simulink model "simL0_multiPath"  (R2024a)
settings: Solver=ode4  StartTime=0.0  StopTime=1500  FixedStep=0.01  MaxStep=0.01  MinStep=10^-3  RelTol=0.01
values from neighbouring files (symbols this model uses):
  MegAWESkite = yaml.ReadYaml('MegAWESkite.yaml',false,true)    [runMain.m]
undefined symbols (not defined in the file or in its folder): actuatorLimit, controllerGains_retraction, controllerGains_traction, DiscIntNeverNeededParam, ENVMT, pathparam, simInit, tetherParams, winchParameter
libraries: simulink x9, slpidlib x9, sharedtransform x3, aerolibutil x3, dspswit3 x2, dspinverses x2, shared6dof x1, simulink_extras x1, dspsigops x1, dspstat3 x1, vrlib x1
(part 1 of 5)
settings Model: Creator=Gian  LastModifiedBy=dylaneijkelhof
settings SolverCC: MaxConsecutiveMinStep=1000000000  AlgebraicLoopSolver=LineSearch  MinimalZcImpactIntegration=on
settings DataIOCC: SaveOperatingPoint=on  SaveOutput=off  SignalLogging=off  DSMLogging=off  SaveTime=off
settings OptimizationCC: LifeSpan=inf
settings DebuggingCC: ReadBeforeWriteMsg=DisableAll  WriteAfterWriteMsg=DisableAll  WriteAfterReadMsg=DisableAll  MultiTaskDSMMsg=none  MultiTaskRateTransMsg=warning  UnconnectedInputMsg=warning  UnconnectedOutputMsg=warning  UnconnectedLineMsg=warning  SFUnexpectedBacktrackingDiag=warning  SFNoUnconditionalDefaultTransitionDiag=warning  SFExecutionAtInitializationDiag=none  ArithmeticOperatorsInVariantConditions=warning
settings ModelReferenceCC: UpdateModelReferenceTargets=IfOutOfDate  EnableRefExpFcnMdlSchedulingChecks=on  ModelReferenceMinAlgLoopOccurrences=on
settings SFSimCC: SFSimEcho=off  SimUseLocalCustomCode=off  CustomCodeUndefinedFunction=UseInterfaceOnly
settings RTWCC: RTWUseLocalCustomCode=off  GPUComputeCapability=3.5
settings CodeAppCC: StateflowObjectComments=on
settings GRTTargetCC: TargetLangStandard=C89/C90 (ANSI)
settings ConfigComp: CovMetricSettings=dw  CovSaveCumulativeToWorkspaceVar=on  CovSaveSingleToWorkspaceVar=on  CovExternalEMLEnable=off

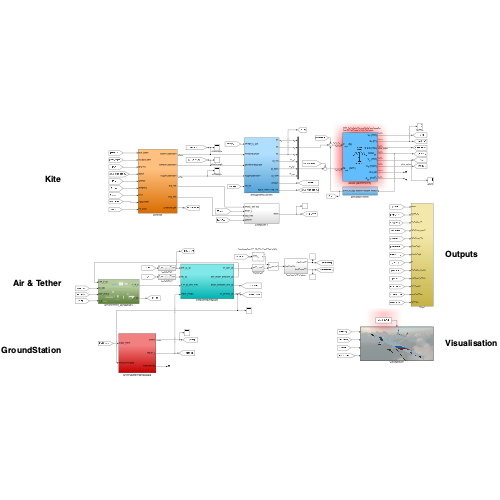
[thumbnail: Simulink's stored preview of the top-level diagram]
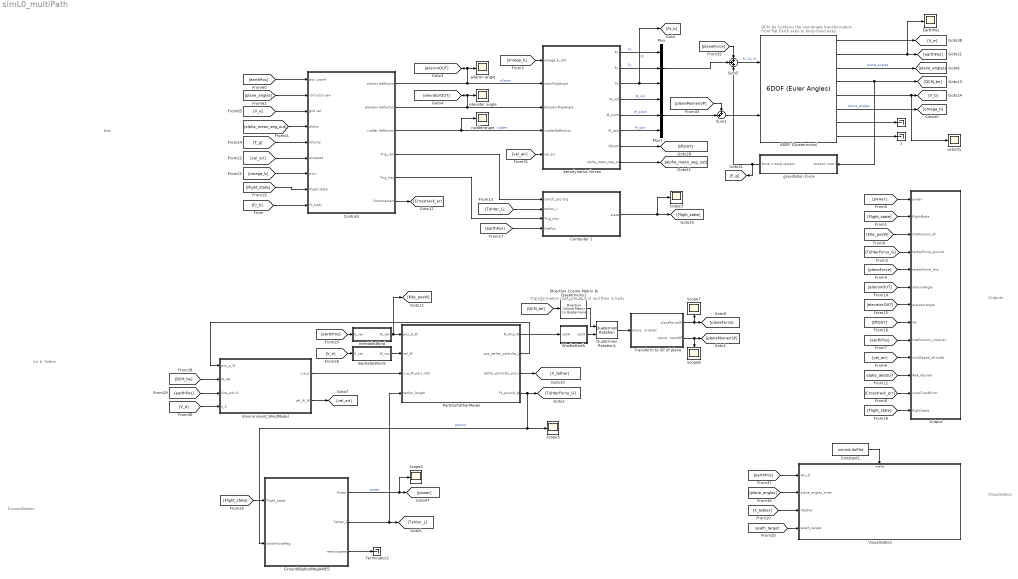
== system simL0_multiPath ==
  note: GroundStation
  note: Transformation of Ft_kite W in O and then in body
  note: DCM_be Contains the coordinate transformation
      | from flat Earth axes to body-fixed axes.
  note: Air & Tether
  note: Kite
  note: Outputs
  note: Visualisation
  "  " : Terminator
  "  1" : Terminator
  6DOF (Quaternions) : shared6dof/6DOF (Euler Angles)  units=Metric (MKS)  mtype=Fixed  rep=Quaternion  xme_0=simInit.pos_O_init  Vm_0=simInit.iniVel  eul_0=simInit.iniEul  pm_0=simInit.bodyRotationRates_init  mass_0=MegAWESkite.mass_aircraft  mass_e=0.5  mass_f=2.0  inertia=MegAWESkite.I_aircraft  inertia_e=eye(3)  inertia_f=2*eye(3)  k_quat=1.0  vre_flag=on  abi_flag=off  aMode=aMode  xme_statename=''  Vm_statename=''  eul_statename=''  quat_statename=''  pm_statename=''  mass_statename=''
  Computer 1 : Subsystem
  Constant1 : Constant  Value=simInit.doPlot
  Controls : Subsystem
  Direction Cosine Matrix to Quaternions1 : sharedtransform/Direction Cosine Matrix  to Quaternions  aMode=aMode  action=None  tolerance=eps(2)
  EarthPos : Scope
  Environment_WindModel : Subsystem
  GroundStationMegAWES : Subsystem
  InertialtoWind : Subsystem
  InertialtoWind1 : Subsystem
  Mux : Mux  Inputs=3
  Mux1 : Mux  Inputs=3
  Output : Subsystem
  ParticleTetherModel : Subsystem
  Quaternion Rotation1 : aerolibutil/Quaternion Rotation
  Scope{2..3,5,7..8} (5 alike) : Scope
  Sum1 : Sum  Inputs=++|
  Sum5 : Sum  Inputs=+++
  Terminator2 : Terminator
  Transform to SP of plane : Subsystem
  Visualisation : Subsystem
      mask Display: image('/Users/dylaneijkelhof/Documents/Matlab/MegAWES/Lib/DE2019_Aircraft.jpeg'); % Use "Edit Image" on toolstrip to change.
  WindtoEarth : Subsystem
  aerodynamic forces : Subsystem
  aileron angle : Scope
  elevator angle : Scope
  gravitation force : Subsystem
  rudderangle : Scope
  velocity : Scope
  wires:
  6DOF (Quaternions)/7 -> "  "/1
  6DOF (Quaternions)/4 -> gravitation force/1(rotation matrix), [DCM_be]
  6DOF (Quaternions)/5 -> velocity/1, [V_b]
  6DOF (Quaternions)/3 -> [plane_angles]  "plane_angles"
  aerodynamic forces/5(M_pitch) -> Mux1/2  "M_pitch"
  aerodynamic forces/6(M_yaw) -> Mux1/3  "M_yaw"
  aerodynamic forces/2(Fy) -> Mux/2  "Fy"
  aerodynamic forces/3(Fz) -> Mux/3, [Fz_b]  "Fz"
  aerodynamic forces/4(M_roll) -> Mux1/1  "M_roll"
  aerodynamic forces/1(Fx) -> Mux/1  "Fx"
  Mux/1 -> Sum5/2
  gravitation force/1(force in body system) -> Sum5/3, [F_g]
  Sum5/1 -> 6DOF (Quaternions)/1  "Fx, Fy, Fz"
  Controls/1(aileron deflection) -> [aileronOUT], aileron angle/1, aerodynamic forces/2(mainFlapAngle)  "aileron"
  Mux1/1 -> Sum1/2
  Sum1/1 -> 6DOF (Quaternions)/2
  6DOF (Quaternions)/1 -> [V_e]
  6DOF (Quaternions)/6 -> [omega_b]  "plane_angles"
  aerodynamic forces/7(liftOUT) -> [liftOUT]
  aerodynamic forces/8(alpha_mean_seg_out) -> [alpha_mean_seg_out]
  [earthPos] -> Controls/1("pos. plane ")
  [plane_angles] -> Controls/2(roll pitch yaw)
  [V_e] -> Controls/3(gnd vel.)
  [alpha_mean_seg_out] -> Controls/4(alpha)
  [vel_air] -> Controls/6(airspeed)
  [omega_b] -> Controls/7(p-q-r)
  [F_g] -> Controls/5(Gravity)
  6DOF (Quaternions)/8 -> "  1"/1
  [omega_b] -> aerodynamic forces/1(omega_b_dist)
  [Fz_b] -> Controls/9("Fz_body ")
  GroundStationMegAWES/3(reeloutspeed) -> Terminator2/1
  6DOF (Quaternions)/2 -> EarthPos/1, [earthPos]
  GroundStationMegAWES/1(Power) -> Scope2/1, [power]  "power"
  Controls/2(elevator deflection) -> aerodynamic forces/3(ElevatorFlapAngle), [elevatorOUT], elevator angle/1
  [Flight_state] -> Controls/8(Flight state)
  [Flight_state] -> GroundStationMegAWES/1(Flight_state)
  ParticleTetherModel/2(pos_tether_particles_W) -> Environment_WindModel/1(pos_p_W)
  [earthPos] -> InertialtoWind/1(E_vec)
  InertialtoWind/1(W_vec) -> [Kite_posW], ParticleTetherModel/1(pos_G_W)
  InertialtoWind1/1(W_vec) -> ParticleTetherModel/2(vel_W)
  [V_e] -> InertialtoWind1/1(E_vec)
  Environment_WindModel/1(v_w_p) -> ParticleTetherModel/3(v_w_W_part_mat)
  GroundStationMegAWES/2(Tether_L) -> ParticleTetherModel/4(tether_length), [Tehter_L]
  [DCM_be] -> Environment_WindModel/2(M_OB)
  [earthPos] -> Environment_WindModel/3(Kite_pos O)
  Environment_WindModel/2(vel_W_W) -> [vel_air]
  [V_b] -> Environment_WindModel/4(v_b)
  Transform to SP of plane/2(planeMomentSP) -> [planeMomenSP], Scope8/1
  Transform to SP of plane/1(planeForceSP) -> [planeForce], Scope7/1
  [vel_air] -> aerodynamic forces/5(vel_air)
  [planeForce] -> Sum5/1
  ParticleTetherModel/4(Ft_ground_W) -> GroundStationMegAWES/2(winchForceMag), Scope5/1, [TehterForce_G]  "ground"
  ParticleTetherModel/1(Ft_Kite_W) -> WindtoEarth/1(vecW)
  Direction Cosine Matrix to Quaternions1/1 -> Quaternion Rotation1/1
  [DCM_be] -> Direction Cosine Matrix to Quaternions1/1
  WindtoEarth/1(vecO) -> Quaternion Rotation1/2
  Quaternion Rotation1/1 -> Transform to SP of plane/1(planeForceVec)
  [planeMomenSP] -> Sum1/1
  ParticleTetherModel/3(tether_particles_pos_W) -> [X_tether]
  [X_tether] -> Visualisation/3(Xtether)
  [plane_angles] -> Visualisation/2(plane_angles_euler)
  [earthPos] -> Visualisation/1(Pos_O)
  Controls/3(rudder deflection) -> rudderangle/1, aerodynamic forces/4(rudderDeflection)  "rudder"
  Controls/6(Crosstrackerr) -> [Crosstrack_err]
  Controls/4(Trig_retr) -> Computer 1/1(switch_pos trig)
  Computer 1/1(state) -> Scope3/1, [Flight_state]
  Controls/5(Trig_trac) -> Computer 1/3(Trig_trac)
  [Tehter_L] -> Computer 1/2(tether_L)
  [earthPos] -> Computer 1/4(kitePos)
  Constant1/1 -> Visualisation/Enable
  [spath_target] -> Visualisation/4(spath_target)
  [Flight_state] -> Output/2(flightMode)
  [Kite_posW] -> Output/3(kitePosition_W)
  [TehterForce_G] -> Output/4(tetherForce_ground)
  [planeForce] -> Output/5(tetherForce_kite)
  [aileronOUT] -> Output/6(aileronAngle)
  [elevatorOUT] -> Output/7(elevatorAngle)
  [liftOUT] -> Output/8(lift)
  [earthPos] -> Output/9(kitePosition_intertial)
  [vel_air] -> Output/10(windSpeed_altitude)
  [alpha_desOUT] -> Output/11(AoA_desired)
  [Crosstrack_err] -> Output/12(crossTrackError)
  [Flight_state] -> Output/13(flightState)
  [power] -> Output/1(power)

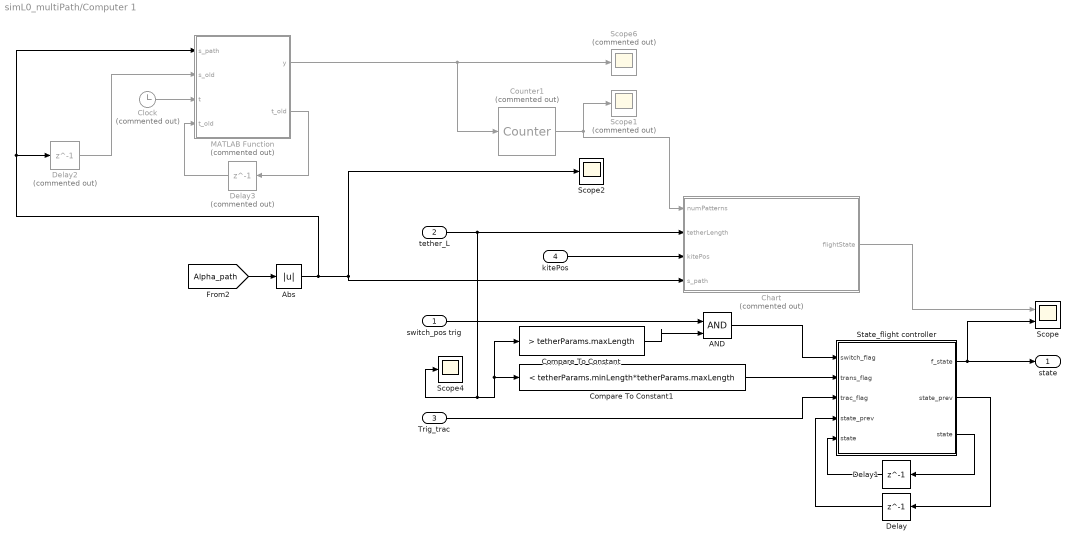
== system simL0_multiPath/Computer 1 ==
  switch_pos trig : Inport
  tether_L : Inport  Port=2
  Trig_trac : Inport  Port=3
  kitePos : Inport  Port=4
  AND : Logic  IconShape=distinctive  AllPortsSameDT=off  OutDataTypeStr=boolean
  Abs : Abs  SaturateOnIntegerOverflow=off
  Chart : Stateflow chart  Commented=on  TreatAsAtomicUnit=on
  Clock : Clock  Commented=on
  Compare To Constant : simulink/Logic and Bit Operations/Compare To Constant  relop=>  const=tetherParams.maxLength  OutDataTypeStr=boolean
  Compare To Constant1 : simulink/Logic and Bit Operations/Compare To Constant  relop=<  const=tetherParams.minLength*tetherParams.maxLength  OutDataTypeStr=boolean
  Counter1 : dspswit3/Counter  Commented=on  Direction=Up  CountEvent=Non-zero sample  CounterSize=User defined  MaxCount=1e9  InitialCount=0  Output=Count  HitValue=32  ResetInput=off  SamplesPerFrame=1  Ts=1  CntDtype=double  HitDtype=Logical
  Delay : Delay  DelayLength=1  InitialCondition=1
  Delay1 : Delay  DelayLength=1  InitialCondition=1
  Delay2 : Delay  Commented=on  DelayLength=1
  Delay3 : Delay  Commented=on  DelayLength=1
  MATLAB Function : MATLAB Function  Commented=on  TreatAsAtomicUnit=on
  Scope : Scope  NumInputPorts=2
  Scope1 : Scope  Commented=on
  Scope2 : Scope
  Scope4 : Scope
  Scope6 : Scope  Commented=on
  State_flight controller : MATLAB Function  TreatAsAtomicUnit=on
  state : Outport
  wires:
  tether_L/1 -> Scope4/1, Compare To Constant/1, Compare To Constant1/1, Chart/2(tetherLength)
  AND/1 -> State_flight controller/1(switch_flag)
  Compare To Constant1/1 -> State_flight controller/2(trans_flag)
  switch_pos trig/1 -> AND/1
  State_flight controller/1(f_state) -> Scope/2, state/1
  Compare To Constant/1 -> AND/2
  Trig_trac/1 -> State_flight controller/3(trac_flag)
  Chart/1(flightState) -> Scope/1
  kitePos/1 -> Chart/3(kitePos)
  [Alpha_path] -> Abs/1
  Delay/1 -> State_flight controller/4("state_prev ")
  State_flight controller/2(state_prev) -> Delay/1
  Delay1/1 -> State_flight controller/5("state ")
  State_flight controller/3(state) -> Delay1/1
  Abs/1 -> MATLAB Function/1(s_path), Delay2/1, Scope2/1, Chart/4(s_path)
  Counter1/1 -> Chart/1(numPatterns), Scope1/1
  Delay2/1 -> MATLAB Function/2(s_old)
  MATLAB Function/1(y) -> Counter1/1, Scope6/1
  MATLAB Function/2(t_old) -> Delay3/1
  Delay3/1 -> MATLAB Function/4("t_old ")
  Clock/1 -> MATLAB Function/3(t)

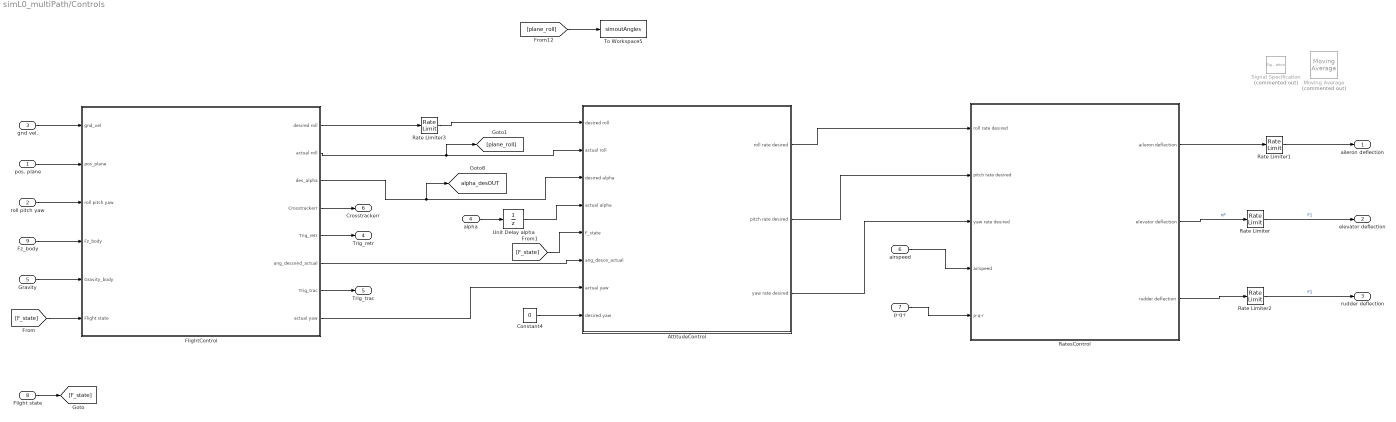
== system simL0_multiPath/Controls ==
  "pos. plane " : Inport
  roll pitch yaw : Inport  Port=2
  gnd vel. : Inport  Port=3
  alpha : Inport  Port=4
  Gravity : Inport  Port=5
  airspeed : Inport  Port=6
  p-q-r : Inport  Port=7
  Flight state : Inport  Port=8
  "Fz_body " : Inport  Port=9
  " FlightControl" : Subsystem
  AttitudeControl : Subsystem
  Constant4 : Constant  Value=0
  Moving Average : dspstat3/Moving Average  Commented=on  Method=Exponential weighting  ForgettingFactorPort=off  SpecifyWindowLength=on  WindowLength=20  OverlapLength=19  AllowArbitraryInputLength=off  ForgettingFactor=0.9  SimulateUsing=Code generation
  Rate Limiter : RateLimiter  RisingSlewLimit=actuatorLimit.rateElevator  FallingSlewLimit=-actuatorLimit.rateElevator  SampleTimeMode=inherited
  Rate Limiter1 : RateLimiter  RisingSlewLimit=actuatorLimit.rateAileron  FallingSlewLimit=-actuatorLimit.rateAileron  SampleTimeMode=inherited
  Rate Limiter2 : RateLimiter  RisingSlewLimit=actuatorLimit.rateElevator  FallingSlewLimit=-actuatorLimit.rateElevator  SampleTimeMode=inherited
  Rate Limiter3 : RateLimiter  RisingSlewLimit=actuatorLimit.rateAileron  FallingSlewLimit=-actuatorLimit.rateAileron  SampleTimeMode=inherited
  RatesControl : Subsystem
  Signal Specification : SignalSpecification  Commented=on  Dimensions=1
  To Workspace5 : ToWorkspace  VariableName=simoutAngles  SaveFormat=Structure With Time  SampleTime=-1
  Unit Delay alpha : UnitDelay  SampleTime=-1  HasFrameUpgradeWarning=on
  aileron deflection : Outport  VectorParamsAs1DForOutWhenUnconnected=off
  elevator deflection : Outport  Port=2  VectorParamsAs1DForOutWhenUnconnected=off
  rudder deflection : Outport  Port=3  VectorParamsAs1DForOutWhenUnconnected=off
  Trig_retr : Outport  Port=4
  Trig_trac : Outport  Port=5
  Crosstrackerr : Outport  Port=6
  tag scope: alpha_desOUT=global
  wires:
  alpha/1 -> Unit Delay alpha/1
  AttitudeControl/1(roll rate desired) -> RatesControl/1(roll rate desired)
  AttitudeControl/2(pitch rate desired) -> RatesControl/2(pitch rate desired)
  p-q-r/1 -> RatesControl/5(p-q-r)
  RatesControl/1(aileron deflection) -> Rate Limiter1/1
  RatesControl/3(rudder deflection) -> Rate Limiter2/1
  Rate Limiter/1 -> elevator deflection/1  "F1"
  Rate Limiter1/1 -> aileron deflection/1
  [plane_roll] -> To Workspace5/1
  gnd vel./1 -> " FlightControl"/1(gnd_vel)
  "pos. plane "/1 -> " FlightControl"/2(pos_plane)
  roll pitch yaw/1 -> " FlightControl"/3(roll pitch yaw)
  " FlightControl"/1(desired roll) -> Rate Limiter3/1
  " FlightControl"/2(actual roll) -> [plane_roll], AttitudeControl/2(actual roll)
  "Fz_body "/1 -> " FlightControl"/4(Fz_body)
  " FlightControl"/3(des_alpha) -> [alpha_desOUT], AttitudeControl/3(desired alpha)
  airspeed/1 -> RatesControl/4(airspeed)
  RatesControl/2(elevator deflection) -> Rate Limiter/1  "nF"
  Gravity/1 -> " FlightControl"/5("Gravity_body ")
  " FlightControl"/5(Trig_retr) -> Trig_retr/1
  Flight state/1 -> [F_state]
  [F_state] -> " FlightControl"/6(Flight state)
  [F_state] -> AttitudeControl/5(F_state)
  " FlightControl"/7(Trig_trac) -> Trig_trac/1
  Unit Delay alpha/1 -> AttitudeControl/4(actual alpha)
  " FlightControl"/4(Crosstrackerr) -> Crosstrackerr/1
  " FlightControl"/6(ang_descend_actual) -> AttitudeControl/6("ang_desce_actual ")
  Rate Limiter2/1 -> rudder deflection/1  "F1"
  " FlightControl"/8(actual yaw) -> AttitudeControl/7(actual yaw)
  Constant4/1 -> AttitudeControl/8(desired yaw)
  AttitudeControl/3(yaw rate desired) -> RatesControl/3(yaw rate desired)
  Rate Limiter3/1 -> AttitudeControl/1(desired roll)

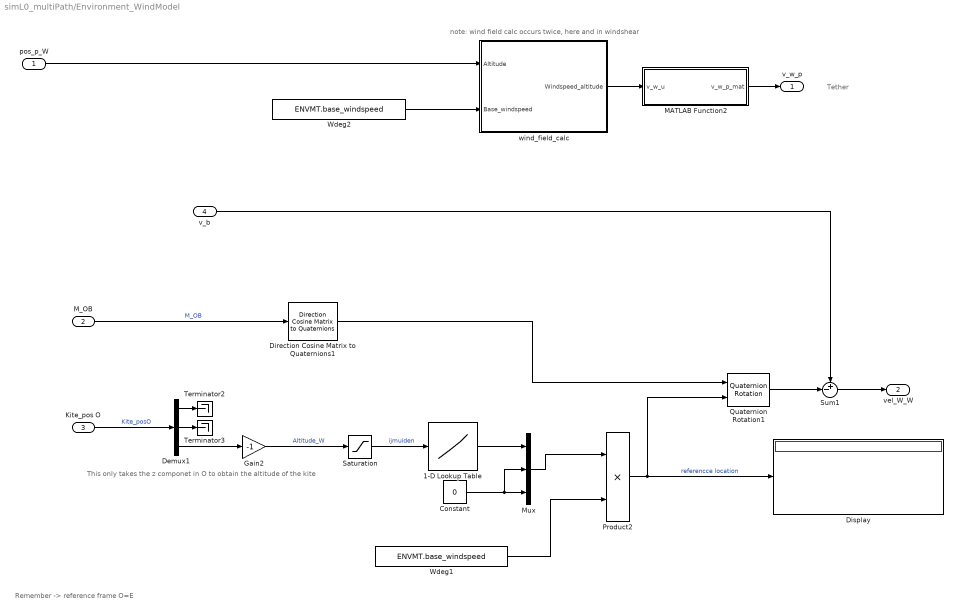
== system simL0_multiPath/Environment_WindModel ==
  note: Tether
  note: note: wind field calc occurs twice, here and in windshear
  note: Remember -> reference frame O=E
  note: This only takes the z componet in O to obtain the altitude of the kite
  pos_p_W : Inport
  M_OB : Inport  Port=2
  Kite_pos O : Inport  Port=3
  v_b : Inport  Port=4
  1-D Lookup Table : Lookup_n-D  NumberOfTableDimensions=1  BreakpointsForDimension1=ENVMT.wind_height  Table=ENVMT.wind_data  InternalRulePriority=Speed  RndMeth=Simplest
  Constant : Constant  Value=0
  Demux1 : Demux  Outputs=3
  Direction Cosine Matrix to Quaternions1 : sharedtransform/Direction Cosine Matrix  to Quaternions  aMode=aMode  action=None  tolerance=eps(2)
  Display : Display
  Gain2 : Gain  Gain=-1
  MATLAB Function2 : MATLAB Function  TreatAsAtomicUnit=on
  Mux : Mux  Inputs=3
  Product2 : Product  InputSameDT=on  SaturateOnIntegerOverflow=on  OutDataTypeStr=Inherit: Same as first input
  Quaternion Rotation1 : aerolibutil/Quaternion Rotation
  Saturation : Saturate  UpperLimit=ENVMT.height_max  LowerLimit=ENVMT.wind_height(1)
  Sum1 : Sum  Inputs=+-|
  Terminator2 : Terminator
  Terminator3 : Terminator
  Wdeg1 : Constant  Value=ENVMT.base_windspeed  OutDataTypeStr=Inherit: Inherit via back propagation
  Wdeg2 : Constant  Value=ENVMT.base_windspeed  OutDataTypeStr=Inherit: Inherit via back propagation
  wind_field_calc : Subsystem
  v_w_p : Outport  VectorParamsAs1DForOutWhenUnconnected=off
  vel_W_W : Outport  Port=2
  wires:
  wind_field_calc/1(Windspeed_altitude) -> MATLAB Function2/1(v_w_u)
  Wdeg2/1 -> wind_field_calc/2(Base_windspeed)
  pos_p_W/1 -> wind_field_calc/1(Altitude)
  MATLAB Function2/1(v_w_p_mat) -> v_w_p/1
  Demux1/1 -> Terminator2/1
  Demux1/3 -> Gain2/1
  Demux1/2 -> Terminator3/1
  Kite_pos O/1 -> Demux1/1  "Kite_posO"
  M_OB/1 -> Direction Cosine Matrix to Quaternions1/1  "M_OB"
  Saturation/1 -> 1-D Lookup Table/1  "ijmuiden"
  Gain2/1 -> Saturation/1  "Altitude_W"
  Wdeg1/1 -> Product2/2
  Product2/1 -> Quaternion Rotation1/2, Display/1  "referencce location"
  Mux/1 -> Product2/1
  Direction Cosine Matrix to Quaternions1/1 -> Quaternion Rotation1/1
  1-D Lookup Table/1 -> Mux/1
  Constant/1 -> Mux/2, Mux/3
  Quaternion Rotation1/1 -> Sum1/2
  Sum1/1 -> vel_W_W/1
  v_b/1 -> Sum1/1

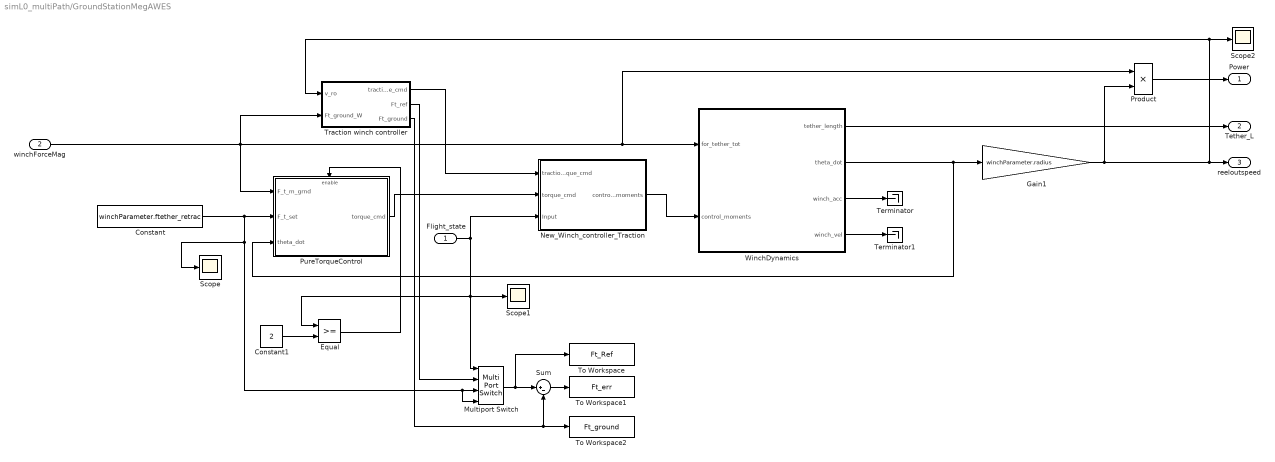
== system simL0_multiPath/GroundStationMegAWES ==
  Flight_state : Inport
  winchForceMag : Inport  Port=2
  " New_Winch_controller_Traction" : Subsystem
  Constant : Constant  Value=winchParameter.ftether_retrac
  Constant1 : Constant  Value=2
  Equal : RelationalOperator  OutDataTypeStr=boolean  RndMeth=Simplest  InputSameDT=off
  Gain1 : Gain  Gain=winchParameter.radius
  Multiport Switch : MultiPortSwitch  SaturateOnIntegerOverflow=off  InputSameDT=off
  Product : Product
  PureTorqueControl : Subsystem
  Scope : Scope
  Scope1 : Scope
  Scope2 : Scope
  Sum : Sum  Inputs=|+-
  Terminator : Terminator
  Terminator1 : Terminator
  To Workspace : ToWorkspace  VariableName=Ft_Ref  SaveFormat=Timeseries  SampleTime=-1
  To Workspace1 : ToWorkspace  VariableName=Ft_err  SaveFormat=Timeseries  SampleTime=-1
  To Workspace2 : ToWorkspace  VariableName=Ft_ground  SaveFormat=Timeseries  SampleTime=-1
  Traction winch controller : Subsystem
  WinchDynamics : Subsystem
  Power : Outport  VectorParamsAs1DForOutWhenUnconnected=off
  Tether_L : Outport  Port=2
  reeloutspeed : Outport  Port=3  VectorParamsAs1DForOutWhenUnconnected=off
  wires:
  WinchDynamics/1(tether_length) -> Tether_L/1
  Gain1/1 -> Traction winch controller/1(v_ro), Scope2/1, reeloutspeed/1, Product/2
  WinchDynamics/4(winch_vel) -> Terminator1/1
  WinchDynamics/3(winch_acc) -> Terminator/1
  WinchDynamics/2(theta_dot) -> PureTorqueControl/3(theta_dot), Gain1/1
  Product/1 -> Power/1
  winchForceMag/1 -> Traction winch controller/2(Ft_ground_W), Product/1, WinchDynamics/1(for_tether_tot), PureTorqueControl/1(F_t_m_grnd)
  Traction winch controller/1(traction_torque_cmd) -> " New_Winch_controller_Traction"/1(traction_torque_cmd)
  " New_Winch_controller_Traction"/1(control_moments) -> WinchDynamics/2(control_moments)
  Constant/1 -> PureTorqueControl/2(F_t_set), Multiport Switch/4, Multiport Switch/3, Scope/1
  Flight_state/1 -> " New_Winch_controller_Traction"/3(Input), Equal/1, Multiport Switch/1, Scope1/1
  Traction winch controller/2(Ft_ref) -> Multiport Switch/2
  Traction winch controller/3(Ft_ground) -> Sum/2, To Workspace2/1
  Multiport Switch/1 -> To Workspace/1, Sum/1
  Sum/1 -> To Workspace1/1
  Constant1/1 -> Equal/2
  Equal/1 -> PureTorqueControl/Enable
  PureTorqueControl/1(torque_cmd) -> " New_Winch_controller_Traction"/2(torque_cmd)

== system simL0_multiPath/InertialtoWind ==
  E_vec : Inport
  Demux : Demux  Outputs=3
  Gain : Gain
  Gain1 : Gain  Gain=-1
  Gain2 : Gain  Gain=-1
  Mux4 : Mux  Inputs=3
  W_vec : Outport
  wires:
  Demux/2 -> Gain1/1
  Demux/1 -> Gain/1
  Gain1/1 -> Mux4/2
  Gain/1 -> Mux4/1
  Gain2/1 -> Mux4/3
  E_vec/1 -> Demux/1
  Mux4/1 -> W_vec/1
  Demux/3 -> Gain2/1

== system simL0_multiPath/InertialtoWind1 ==
  E_vec : Inport
  Demux : Demux  Outputs=3
  Gain : Gain
  Gain1 : Gain  Gain=-1
  Gain2 : Gain  Gain=-1
  Mux4 : Mux  Inputs=3
  W_vec : Outport
  wires:
  Demux/2 -> Gain1/1
  Demux/1 -> Gain/1
  Gain1/1 -> Mux4/2
  Gain/1 -> Mux4/1
  Gain2/1 -> Mux4/3
  E_vec/1 -> Demux/1
  Mux4/1 -> W_vec/1
  Demux/3 -> Gain2/1

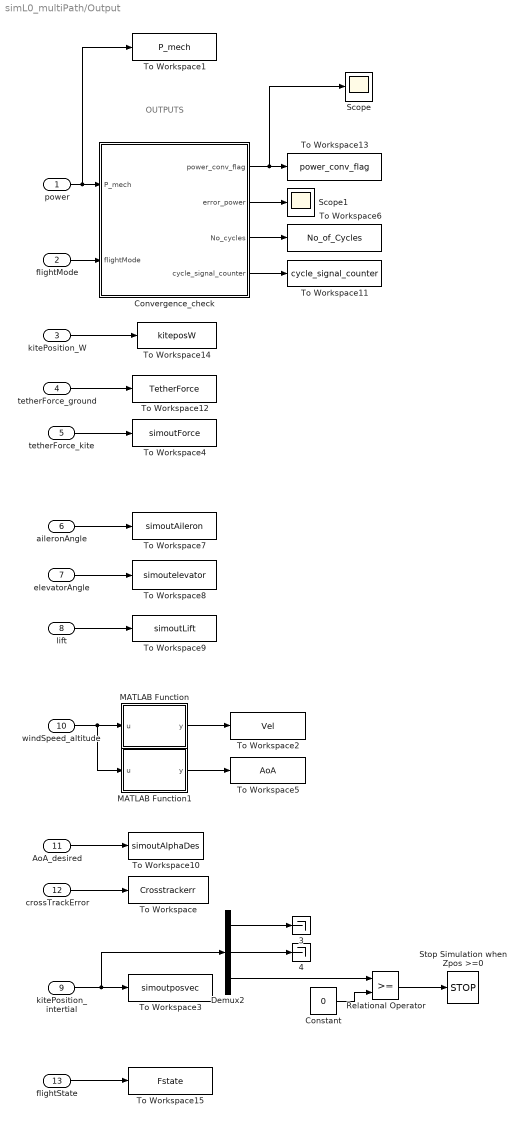
== system simL0_multiPath/Output ==
  note: OUTPUTS
  power : Inport
  flightMode : Inport  Port=2
  kitePosition_W : Inport  Port=3
  tetherForce_ground : Inport  Port=4
  tetherForce_kite : Inport  Port=5
  aileronAngle : Inport  Port=6
  elevatorAngle : Inport  Port=7
  lift : Inport  Port=8
  kitePosition_intertial : Inport  Port=9
  windSpeed_altitude : Inport  Port=10
  AoA_desired : Inport  Port=11
  crossTrackError : Inport  Port=12
  flightState : Inport  Port=13
  "  3" : Terminator
  "  4" : Terminator
  Constant : Constant  Value=0
  Convergence_check : Subsystem
  Demux2 : Demux  Outputs=3
  MATLAB Function : MATLAB Function  TreatAsAtomicUnit=on
  MATLAB Function1 : MATLAB Function  TreatAsAtomicUnit=on
  Relational Operator : RelationalOperator  OutDataTypeStr=boolean  RndMeth=Simplest  InputSameDT=off
  Scope : Scope
  Scope1 : Scope
  Stop Simulation when Zpos >=0 : Stop
  To Workspace : ToWorkspace  VariableName=Crosstrackerr  SaveFormat=Timeseries  SampleTime=-1
  To Workspace1 : ToWorkspace  VariableName=P_mech  SaveFormat=Timeseries  SampleTime=0.01
  To Workspace10 : ToWorkspace  VariableName=simoutAlphaDes  SaveFormat=Timeseries  SampleTime=-1
  To Workspace11 : ToWorkspace  VariableName=cycle_signal_counter  SaveFormat=Timeseries  SampleTime=-1
  To Workspace12 : ToWorkspace  VariableName=TetherForce  SaveFormat=Timeseries  SampleTime=-1
  To Workspace13 : ToWorkspace  VariableName=power_conv_flag  SampleTime=-1
      settings: MaxDataPoints=1
  To Workspace14 : ToWorkspace  VariableName=kiteposW  SaveFormat=Timeseries  SampleTime=0.01
  To Workspace15 : ToWorkspace  VariableName=Fstate  SaveFormat=Timeseries  SampleTime=0.01
  To Workspace2 : ToWorkspace  VariableName=Vel  SaveFormat=Timeseries  SampleTime=-1
  To Workspace3 : ToWorkspace  VariableName=simoutposvec  SaveFormat=Timeseries  SampleTime=-1
  To Workspace4 : ToWorkspace  VariableName=simoutForce  SaveFormat=Timeseries  SampleTime=-1
  To Workspace5 : ToWorkspace  VariableName=AoA  SaveFormat=Timeseries  SampleTime=-1
  To Workspace6 : ToWorkspace  VariableName=No_of_Cycles  SampleTime=-1
      settings: MaxDataPoints=1
  To Workspace7 : ToWorkspace  VariableName=simoutAileron  SaveFormat=Timeseries  SampleTime=-1
  To Workspace8 : ToWorkspace  VariableName=simoutelevator  SaveFormat=Timeseries  SampleTime=-1
  To Workspace9 : ToWorkspace  VariableName=simoutLift  SaveFormat=Timeseries  SampleTime=-1
  wires:
  power/1 -> To Workspace1/1, Convergence_check/1(P_mech)
  lift/1 -> To Workspace9/1
  kitePosition_intertial/1 -> Demux2/1, To Workspace3/1
  tetherForce_ground/1 -> To Workspace12/1
  flightState/1 -> To Workspace15/1
  aileronAngle/1 -> To Workspace7/1
  crossTrackError/1 -> To Workspace/1
  MATLAB Function/1(y) -> To Workspace2/1
  tetherForce_kite/1 -> To Workspace4/1
  Convergence_check/4(cycle_signal_counter) -> To Workspace11/1
  Convergence_check/3(No_cycles) -> To Workspace6/1
  MATLAB Function1/1(y) -> To Workspace5/1
  Constant/1 -> Relational Operator/2
  Convergence_check/1(power_conv_flag) -> To Workspace13/1, Scope/1
  Demux2/3 -> Relational Operator/1
  elevatorAngle/1 -> To Workspace8/1
  flightMode/1 -> Convergence_check/2(flightMode)
  windSpeed_altitude/1 -> MATLAB Function1/1(u), MATLAB Function/1(u)
  Relational Operator/1 -> Stop Simulation when Zpos >=0/1
  AoA_desired/1 -> To Workspace10/1
  Demux2/2 -> "  4"/1
  Convergence_check/2(error_power) -> Scope1/1
  kitePosition_W/1 -> To Workspace14/1
  Demux2/1 -> "  3"/1

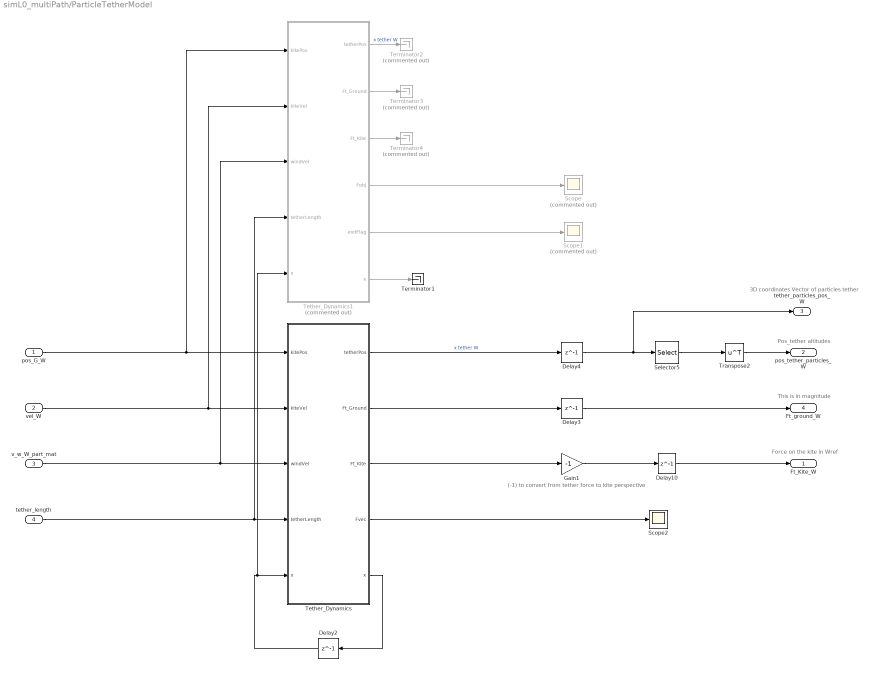
== system simL0_multiPath/ParticleTetherModel ==
  note: 3D coordinates Vector of particles tether
  note: Pos_tether altitudes
  note: Force on the kite in Wref
  note: This is in magnitude
  note: (-1) to convert from tether force to kite perspective
  pos_G_W : Inport
  vel_W : Inport  Port=2
  v_w_W_part_mat : Inport  Port=3
  tether_length : Inport  Port=4
  Delay10 : Delay  DelayLength=1  InitialCondition=zeros(3,1)
  Delay2 : Delay  DelayLength=1  InitialCondition=tetherParams.Tn_vect
  Delay3 : Delay  DelayLength=1
  Delay4 : Delay  DelayLength=1  InitialCondition=tetherParams.pos_p_init
  Gain1 : Gain  Gain=-1
  Scope : Scope  Commented=on
  Scope1 : Scope  Commented=on
  Scope2 : Scope
  Selector5 : Selector  NumberOfDimensions=2  InputPortWidth=3  IndexOptions=Index vector (dialog),Select all  Indices=3,1  OutputSizes=1,1
  Terminator1 : Terminator
  Terminator2 : Terminator  Commented=on
  Terminator3 : Terminator  Commented=on
  Terminator4 : Terminator  Commented=on
  Tether_Dynamics : MATLAB Function  TreatAsAtomicUnit=on
  Tether_Dynamics1 : MATLAB Function  Commented=on  TreatAsAtomicUnit=on
  Transpose2 : Math  Operator=transpose
  Ft_Kite_W : Outport  VectorParamsAs1DForOutWhenUnconnected=off
  pos_tether_particles_W : Outport  Port=2  VectorParamsAs1DForOutWhenUnconnected=off
  tether_particles_pos_W : Outport  Port=3
  Ft_ground_W : Outport  Port=4  VectorParamsAs1DForOutWhenUnconnected=off
  wires:
  Selector5/1 -> Transpose2/1
  Transpose2/1 -> pos_tether_particles_W/1
  Delay4/1 -> tether_particles_pos_W/1, Selector5/1
  Delay3/1 -> Ft_ground_W/1
  Delay10/1 -> Ft_Kite_W/1
  Tether_Dynamics1/4(Fobj) -> Scope/1
  tether_length/1 -> Tether_Dynamics1/4(tetherLength), Tether_Dynamics/4(tetherLength)
  Gain1/1 -> Delay10/1
  Delay2/1 -> Tether_Dynamics1/5("x "), Tether_Dynamics/5("x ")
  v_w_W_part_mat/1 -> Tether_Dynamics1/3(windVel), Tether_Dynamics/3(windVel)
  pos_G_W/1 -> Tether_Dynamics1/1(kitePos), Tether_Dynamics/1(kitePos)
  vel_W/1 -> Tether_Dynamics1/2(kiteVel), Tether_Dynamics/2(kiteVel)
  Tether_Dynamics1/5(exitFlag) -> Scope1/1
  Tether_Dynamics1/1(tetherPos) -> Terminator2/1  "x tether W"
  Tether_Dynamics1/2(Ft_Ground) -> Terminator3/1
  Tether_Dynamics1/3(Ft_Kite) -> Terminator4/1
  Tether_Dynamics1/6(x) -> Terminator1/1
  Tether_Dynamics/1(tetherPos) -> Delay4/1  "x tether W"
  Tether_Dynamics/2(Ft_Ground) -> Delay3/1
  Tether_Dynamics/3(Ft_Kite) -> Gain1/1
  Tether_Dynamics/4(Fvec) -> Scope2/1
  Tether_Dynamics/5(x) -> Delay2/1

== system simL0_multiPath/Transform to SP of plane ==
  planeForceVec : Inport
  Constant : Constant  Value=tetherParams.attachmentPoint_from_cog
  Cross Product : vrlib/Utilities/Cross Product
  planeForceSP : Outport  VectorParamsAs1DForOutWhenUnconnected=off
  planeMomentSP : Outport  Port=2  VectorParamsAs1DForOutWhenUnconnected=off
  wires:
  planeForceVec/1 -> Cross Product/2, planeForceSP/1
  Constant/1 -> Cross Product/1
  Cross Product/1 -> planeMomentSP/1

== system simL0_multiPath/Visualisation ==
  Pos_O : Inport
  plane_angles_euler : Inport  Port=2
  Xtether : Inport  Port=3
  spath_target : Inport  Port=4
  Enable : EnablePort
  Clock : Clock
  Constant : Constant  Value=simInit.sample_time_vis
  Selector : Selector  NumberOfDimensions=2  InputPortWidth=3  IndexOptions=Index vector (dialog),Select all  Indices=1,1  OutputSizes=1,1
  Selector4 : Selector  NumberOfDimensions=2  InputPortWidth=3  IndexOptions=Index vector (dialog),Select all  Indices=2,1  OutputSizes=1,1
  Selector5 : Selector  NumberOfDimensions=2  InputPortWidth=3  IndexOptions=Index vector (dialog),Select all  Indices=3,1  OutputSizes=1,1
  Transpose : Math  Operator=transpose
  Transpose1 : Math  Operator=transpose
  Transpose2 : Math  Operator=transpose
  Visualisation : MATLAB Function  TreatAsAtomicUnit=on
  wires:
  Pos_O/1 -> Visualisation/5(pos_O)
  Clock/1 -> Visualisation/1(t)
  plane_angles_euler/1 -> Visualisation/6(eta_OB)
  Constant/1 -> Visualisation/7(sampletime)
  Selector4/1 -> Transpose1/1
  Selector5/1 -> Transpose2/1
  Transpose/1 -> Visualisation/2(p_t_x)
  Selector/1 -> Transpose/1
  Transpose2/1 -> Visualisation/4(p_t_z)
  Transpose1/1 -> Visualisation/3(p_t_y)
  Xtether/1 -> Selector5/1, Selector4/1, Selector/1
  spath_target/1 -> Visualisation/8(starget)

== system simL0_multiPath/WindtoEarth ==
  vecW : Inport
  Demux : Demux  Outputs=3
  Gain : Gain
  Gain1 : Gain  Gain=-1
  Gain2 : Gain  Gain=-1
  Mux5 : Mux  Inputs=3
  vecO : Outport
  wires:
  Gain1/1 -> Mux5/2
  Demux/2 -> Gain1/1
  Demux/1 -> Gain/1
  Mux5/1 -> vecO/1
  Gain2/1 -> Mux5/3
  vecW/1 -> Demux/1
  Gain/1 -> Mux5/1
  Demux/3 -> Gain2/1

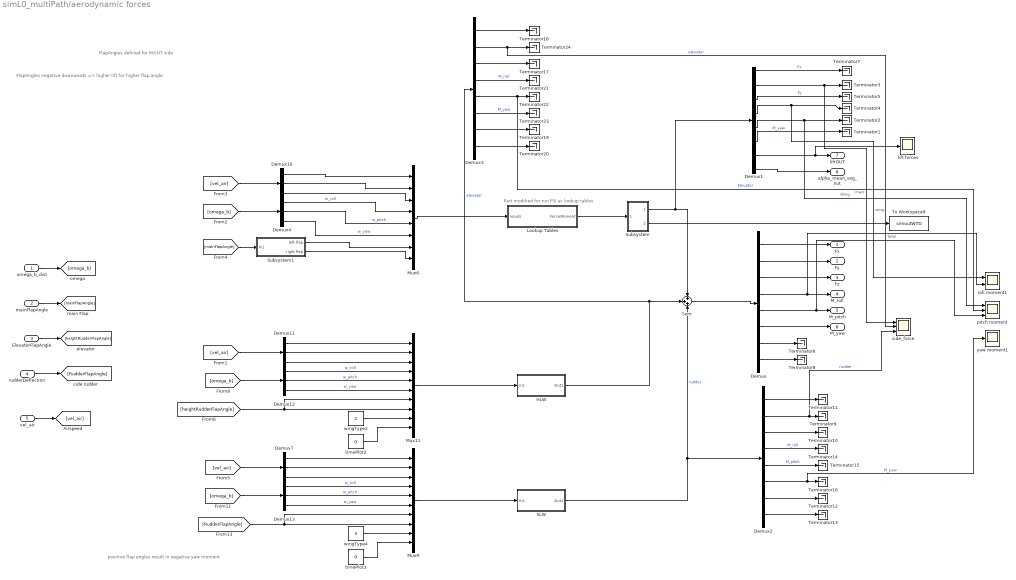
== system simL0_multiPath/aerodynamic forces ==
  note: Part modified for run FSI as lookup tables
  note: positive flap angles result in negative yaw moment
  note: FlapAngles defined for RIGHT side
  note: FlapAngles negative downwards => higher lift for higher flap angle
  omega_b_dist : Inport
  mainFlapAngle : Inport  Port=2
  ElevatorFlapAngle : Inport  Port=3
  rudderDeflection : Inport  Port=4
  vel_air : Inport  Port=5
  Demux{,1..3} (4 alike) : Demux  Outputs=8
  Demux{4,7,10..13} (6 alike) : Demux  Outputs=3
  HLW : Subsystem
  Lookup Tables : Subsystem
  Mux11 : Mux  Inputs=10
  Mux6 : Mux  Inputs=8
  Mux9 : Mux  Inputs=10
  SLW : Subsystem
  Subsystem : Subsystem
  Subsystem1 : Subsystem
  Sum : Sum  Inputs=+++
  Terminator{1..24} (24 alike) : Terminator
  To Workspace9 : ToWorkspace  VariableName=simoutWTD  SaveFormat=Structure With Time  SampleTime=-1
  lift forces : Scope
  pitch moment : Scope  NumInputPorts=3
  roll moment1 : Scope  NumInputPorts=2
  side_force : Scope  NumInputPorts=3
  timePlot2 : Constant  Value=0
  timePlot3 : Constant  Value=0
  wingType2 : Constant  Value=2
  wingType4 : Constant  Value=3
  yaw moment1 : Scope
  Fx : Outport  VectorParamsAs1DForOutWhenUnconnected=off
  Fy : Outport  Port=2  VectorParamsAs1DForOutWhenUnconnected=off
  Fz : Outport  Port=3  VectorParamsAs1DForOutWhenUnconnected=off
  M_roll : Outport  Port=4  VectorParamsAs1DForOutWhenUnconnected=off
  M_pitch : Outport  Port=5  VectorParamsAs1DForOutWhenUnconnected=off
  M_yaw : Outport  Port=6  VectorParamsAs1DForOutWhenUnconnected=off
  liftOUT : Outport  Port=7  VectorParamsAs1DForOutWhenUnconnected=off
  alpha_mean_seg_out : Outport  Port=8  VectorParamsAs1DForOutWhenUnconnected=off
  wires:
  Sum/1 -> Demux/1
  Demux/1 -> Fx/1
  Demux/2 -> Fy/1
  Demux/3 -> Fz/1
  Demux/4 -> roll moment1/2, M_roll/1  "total"
  Demux/5 -> pitch moment/3, M_pitch/1
  Demux1/1 -> Terminator7/1  "Fx"
  Demux1/2 -> side_force/1, Terminator3/1  "main"
  Demux1/3 -> Terminator5/1  "Fz"
  Demux1/4 -> roll moment1/1, Terminator4/1  "wing"
  Demux1/5 -> pitch moment/1, Terminator2/1  "Wing"
  Demux1/6 -> Terminator1/1  "M_yaw"
  Mux6/1 -> Lookup Tables/1(Inputs)
  Demux4/2 -> Mux6/5  "w_pitch"
  Demux4/1 -> Mux6/4  "w_roll"
  Demux4/3 -> Mux6/6  "w_yaw"
  Mux11/1 -> HLW/1(In1)
  omega_b_dist/1 -> [omega_b]
  [omega_b] -> Demux4/1
  mainFlapAngle/1 -> [mainFlapAngle]
  Demux10/1 -> Mux6/1
  Demux10/2 -> Mux6/2
  Demux10/3 -> Mux6/3
  ElevatorFlapAngle/1 -> [heightRudderFlapAngle]
  Demux12/2 -> Mux11/5  "w_pitch"
  Demux12/1 -> Mux11/4  "w_roll"
  Demux12/3 -> Mux11/6  "w_yaw"
  [omega_b] -> Demux12/1
  Demux11/1 -> Mux11/1
  Demux11/2 -> Mux11/2
  wingType2/1 -> Mux11/9
  timePlot2/1 -> Mux11/10
  Demux13/2 -> Mux9/5  "w_pitch"
  Demux13/1 -> Mux9/4  "w_roll"
  Demux13/3 -> Mux9/6  "w_yaw"
  [vel_air] -> Demux7/1
  Demux7/1 -> Mux9/1
  Demux7/2 -> Mux9/2
  Demux7/3 -> Mux9/3
  [RudderFlapAngle] -> Mux9/8, Mux9/7
  wingType4/1 -> Mux9/9
  timePlot3/1 -> Mux9/10
  rudderDeflection/1 -> [RudderFlapAngle]
  Mux9/1 -> SLW/1(In1)
  [omega_b] -> Demux13/1
  Demux11/3 -> Mux11/3
  Subsystem1/1(left flap) -> Mux6/7
  Subsystem1/2(right flap) -> Mux6/8
  [mainFlapAngle] -> Subsystem1/1(In1)
  Demux/7 -> Terminator6/1
  [heightRudderFlapAngle] -> Mux11/8, Mux11/7
  Demux1/7 -> lift forces/1, liftOUT/1
  Demux1/8 -> alpha_mean_seg_out/1
  Demux/8 -> Terminator8/1
  vel_air/1 -> [vel_air]
  [vel_air] -> Demux11/1
  [vel_air] -> Demux10/1
  Demux/6 -> M_yaw/1
  SLW/1(Out1) -> Demux2/1, Sum/3  "rudder"
  Demux2/1 -> Terminator11/1
  Demux2/2 -> side_force/3, Terminator9/1  "rudder"
  Demux2/3 -> Terminator10/1
  Demux2/7 -> Terminator12/1
  Demux2/8 -> Terminator13/1
  Demux2/4 -> Terminator14/1  "M_roll"
  Demux2/5 -> Terminator15/1  "M_pitch"
  Demux2/6 -> yaw moment1/1, Terminator16/1  "M_yaw"
  Demux3/8 -> Terminator20/1
  Demux3/7 -> Terminator19/1
  Demux3/2 -> side_force/2, Terminator24/1  "elevator"
  Demux3/6 -> Terminator23/1  "M_yaw"
  Demux3/5 -> pitch moment/2, Terminator22/1  "Elevator"
  Demux3/3 -> Terminator17/1
  Demux3/4 -> Terminator21/1  "M_roll"
  Demux3/1 -> Terminator18/1
  HLW/1(Out1) -> Sum/2, Demux3/1  "elevator"
  Subsystem/1(Out1) -> Demux1/1, Sum/1
  Subsystem/2(Out2) -> To Workspace9/1
  Lookup Tables/1(ForceMoment) -> Subsystem/1(In1)

== system simL0_multiPath/gravitation force ==
  rotation matrix : Inport
  Constant1 : Constant  Value=[0,0,MegAWESkite.mass_aircraft]
  Direction Cosine Matrix to Quaternions : sharedtransform/Direction Cosine Matrix  to Quaternions  aMode=aMode  action=None  tolerance=eps(2)
  Gain : Gain  Gain=ENVMT.g
  Quaternion Rotation : aerolibutil/Quaternion Rotation
  force in body system : Outport  VectorParamsAs1DForOutWhenUnconnected=off
  wires:
  Direction Cosine Matrix to Quaternions/1 -> Quaternion Rotation/1
  Quaternion Rotation/1 -> force in body system/1
  rotation matrix/1 -> Direction Cosine Matrix to Quaternions/1
  Constant1/1 -> Gain/1
  Gain/1 -> Quaternion Rotation/2

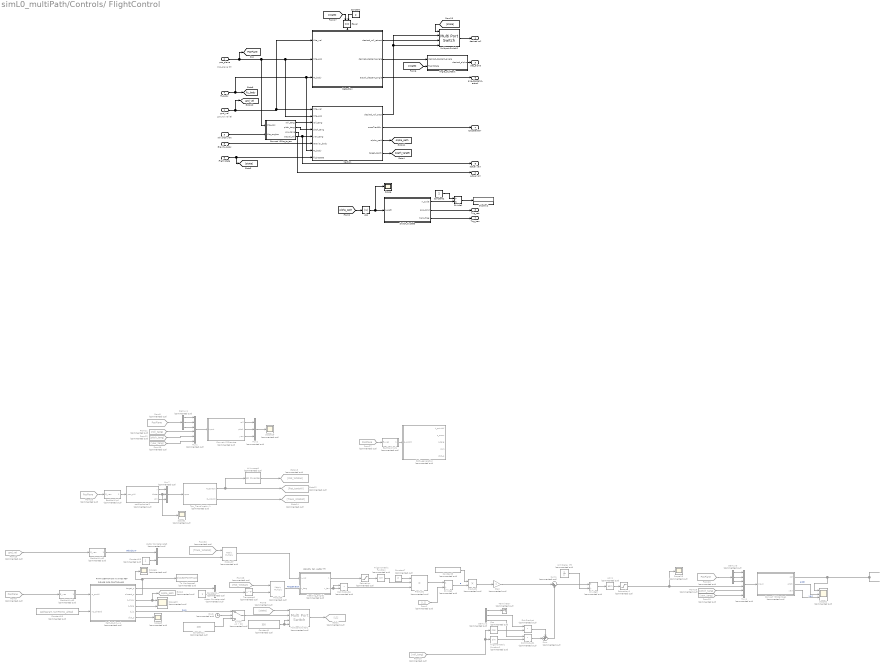
== system simL0_multiPath/Controls/ FlightControl ==
  note: Pos_plane (E)
  note: ground vel (E)
  note: PATH DEFINITION IN WIND REF
  note: Velocity tan vector (T)
  note: FIGURE OF8 CONTROLLER
  gnd_vel : Inport
  pos_plane : Inport  Port=2
  roll pitch yaw : Inport  Port=3
  Fz_body : Inport  Port=4
  "Gravity_body " : Inport  Port=5
  Flight state : Inport  Port=6
  " LU Inverse1" : dspinverses/ LU Inverse  Commented=on
  Abs : Abs  SaturateOnIntegerOverflow=off
  Angle_of_Attack : Subsystem
  Asin1 : Trigonometry  Commented=on  Operator=asin
  Clock : Clock  Commented=on
  Constant : Constant  Value=2
  Constant1 : Constant  Commented=on  Value=350
  Constant11 : Constant  Commented=on  Value=200
  Constant13 : Constant  Commented=on
  Constant14 : Constant  Commented=on
  Constant15 : Constant  Commented=on  Value=pathparam.numPoints_ahead
  Constant2 : Constant  Value=2
  Constant7 : Constant  Commented=on  Value=2
  Constant8 : Constant  Commented=on  Value=MegAWESkite.mass_aircraft
  Convert YPR-e_to_tan : Subsystem
  Convert YPR-tantoe : MATLAB Function  Commented=on  TreatAsAtomicUnit=on
  Convert YPR-tantoe1 : MATLAB Function  Commented=on  TreatAsAtomicUnit=on
  Cos : Trigonometry  Commented=on  Operator=cos
  Demux1 : Demux  Commented=on  Outputs=3
  Demux2 : Demux  Commented=on  Outputs=3
  Demux3 : Demux  Commented=on  Outputs=3
  Display2 : Display
  Divide1 : Product  Inputs=/*
  Divide2 : Product  Commented=on  Inputs=*/
  Divide3 : Product  Commented=on  Inputs=*/
  Dot Product : DotProduct  Commented=on  OutDataTypeStr=Inherit: Inherit via internal rule
  Dot Product1 : DotProduct  Commented=on  OutDataTypeStr=Inherit: Inherit via internal rule
  Dot Product4 : DotProduct  Commented=on  OutDataTypeStr=Inherit: Inherit via internal rule
  EarthtoWind : Subsystem  Commented=on
  EarthtoWind1 : Subsystem  Commented=on
  EarthtoWind2 : Subsystem  Commented=on
  EarthtoWind3 : Subsystem  Commented=on
  Equal : RelationalOperator  Operator===  OutDataTypeStr=boolean  RndMeth=Simplest  InputSameDT=off
  From1 : From  Commented=on  GotoTag=L1
  From10 : From  Commented=on  GotoTag=roll_tang
  From11 : From  Commented=on  GotoTag=roll_tang
  From12 : From  Commented=on  GotoTag=pitch_tang
  From16 : From  Commented=on  GotoTag=yaw_tang
  From18 : From  Commented=on  GotoTag=pitch_tang
  From19 : From  Commented=on  GotoTag=yaw_tang
  From{8..9,20,26} (4 alike) : From  Commented=on  GotoTag=PosPlane  TagVisibility=global
  From27 : From  Commented=on  GotoTag=PosPlane
  From28 : From  Commented=on  GotoTag=Rot_Wtotan
  From29 : From  Commented=on  GotoTag=gnd_vel  TagVisibility=global
  From30 : From  Commented=on  GotoTag=Trans_WtoRot
  From5 : From  Commented=on  GotoTag=state
  Gain : Gain  Commented=on
  Goto1 : Goto  Commented=on  GotoTag=L1
  Goto12 : Goto  Commented=on  GotoTag=Rot_tantoW
  Goto13 : Goto  Commented=on  GotoTag=Rot_Wtotan
  Goto14 : Goto  Commented=on  GotoTag=Trans_WtoRot
  Goto2 : Goto  Commented=on  GotoTag=Alpha_path  TagVisibility=global
  Heading_angle1 : MATLAB Function  Commented=on  TreatAsAtomicUnit=on
  Multiport Switch1 : MultiPortSwitch  Commented=on  DiagnosticForDefault=None  SaturateOnIntegerOverflow=off  InputSameDT=off
  Multiport Switch2 : MultiPortSwitch  DiagnosticForDefault=None  SaturateOnIntegerOverflow=off  InputSameDT=off
  Mux1 : Mux  Commented=on  Inputs=6
  Mux2 : Mux  Commented=on  Inputs=3
  Mux4 : Mux  Commented=on  Inputs=6
  Mux7 : Mux  Commented=on  Inputs=3
  Path_8_sim_v4 : MATLAB Function  Commented=on  TreatAsAtomicUnit=on  SystemSampleTime=0.05
  Path_generation : MATLAB Function  Commented=on  TreatAsAtomicUnit=on  SystemSampleTime=0.01
  Product1 : Product  Commented=on  Inputs=3
  Product2 : Product  Commented=on
  Product6 : Product  Commented=on  Multiplication=Matrix(*)
  Product7 : Product  Commented=on  Multiplication=Matrix(*)
  Retraction : Subsystem
  Saturation : Saturate  Commented=on  UpperLimit=pi/4  LowerLimit=-pi/4
  Saturation1 : Saturate  Commented=on  UpperLimit=1  LowerLimit=-1
  Scope : Scope
  Scope{1,5..6,18..19} (5 alike) : Scope  Commented=on
  Scope2 : Scope  Commented=on  NumInputPorts=3
  Scope23 : Scope  Commented=on  NumInputPorts=2
  Sum : Sum  Commented=on  Inputs=++|
  Sum1 : Sum  Commented=on  Inputs=|++
  Switch : Switch  Commented=on  Criteria=u2 > Threshold  Threshold=20  SaturateOnIntegerOverflow=off  InputSameDT=off
  Switch_flystate : Subsystem
  Tan_Transf matrix 1 : MATLAB Function  Commented=on  TreatAsAtomicUnit=on
  Terminator : Terminator  Commented=on
  To Workspace1 : ToWorkspace  Commented=on  VariableName=ClosestPointTrack  SaveFormat=Timeseries  SampleTime=-1
  Transpose1 : Math  Commented=on  Operator=transpose
  Trigonometric Function : Trigonometry  Commented=on
  Trigonometric Function1 : Trigonometry  Commented=on
  Unit Delay lift : UnitDelay  Commented=on  InitialCondition=1  SampleTime=-1  HasFrameUpgradeWarning=on
  Vector Concatenate1 : Concatenate  Commented=on
  Vector Concatenate3 : Concatenate  Commented=on
  cart2spherical1 : MATLAB Function  Commented=on  TreatAsAtomicUnit=on
  traction : Subsystem
  desired roll : Outport
  actual roll : Outport  Port=2
  des_alpha : Outport  Port=3
  Crosstrackerr : Outport  Port=4
  Trig_retr : Outport  Port=5
  ang_descend_actual : Outport  Port=6
  Trig_trac : Outport  Port=7
  actual yaw : Outport  Port=8
  tag scope: Alpha_path=global, Fz_body=global, PosPlane=global, gnd_vel=global, spath_target=global
  wires:
  gnd_vel/1 -> [gnd_vel], traction/1(Kite_vel), Retraction/1(Kite_vel)
  pos_plane/1 -> [PosPlane], traction/2(Kite_pos), Retraction/2(Kite_pos), Convert YPR-e_to_tan/1(kite_pos)
  Fz_body/1 -> [Fz_body], traction/7(Fz_body), Retraction/3(Fz_body)
  "Gravity_body "/1 -> traction/6(Gravity_body)
  Flight state/1 -> [state], traction/8(flightState)
  [state] -> Multiport Switch2/1
  Demux1/2 -> Mux1/2
  Demux1/1 -> Mux1/1
  Demux1/3 -> Mux1/3
  From8/1 -> Demux1/1
  Mux1/1 -> Convert YPR-tantoe/1(input)
  From11/1 -> Mux1/4
  Convert YPR-tantoe/1(roll) -> Mux2/1
  Convert YPR-tantoe/2(pitch) -> Mux2/2
  Convert YPR-tantoe/3(yaw) -> Mux2/3
  Mux2/1 -> Scope19/1
  From12/1 -> Mux1/5
  From16/1 -> Mux1/6
  cart2spherical1/2(theta) -> Scope1/1, Mux7/2
  cart2spherical1/1(r) -> Mux7/1
  Tan_Transf matrix 1/1(R_tantow) -> Goto12/1, " LU Inverse1"/1
  cart2spherical1/3(phi) -> Mux7/3
  Mux7/1 -> Tan_Transf matrix 1/1(cpos)
  From26/1 -> EarthtoWind/1(E_vec)
  EarthtoWind/1(W_vec) -> cart2spherical1/1(pos_aW)
  " LU Inverse1"/1 -> Goto13/1
  Tan_Transf matrix 1/2(R_wtorot) -> Goto14/1
  From27/1 -> EarthtoWind1/1(E_vec)
  EarthtoWind1/1(W_vec) -> Path_generation/1(a_posW)
  [Alpha_path] -> Abs/1
  Switch_flystate/1(n_cycle) -> Divide1/2
  Switch_flystate/2(pos_cond) -> Trig_retr/1
  Abs/1 -> Scope/1, Switch_flystate/1(s_path)
  Switch_flystate/3(trans_flag) -> Trig_trac/1
  Divide1/1 -> Display2/1
  Constant2/1 -> Divide1/1
  Retraction/3(actual_descent_angle) -> ang_descend_actual/1
  Retraction/1(desired_roll_retract) -> Multiport Switch2/3
  Equal/1 -> Retraction/Enable
  Constant/1 -> Equal/2
  Multiport Switch2/1 -> desired roll/1
  Demux2/3 -> Dot Product1/1
  Constant13/1 -> Vector Concatenate3/2
  Convert YPR-tantoe1/3(yaw) -> Scope2/3  "yaw"
  Heading_angle1/2(v_tan) -> Dot Product4/1, Dot Product4/2
  Dot Product/1 -> Sum/1
  Constant8/1 -> Product2/1
  Convert YPR-tantoe1/1(roll) -> Scope2/1
  Trigonometric Function/1 -> Product1/2
  Path_8_sim_v4/3(s_cnew) -> Scope23/1, Goto2/1
  Path_8_sim_v4/4(s_targ) -> Scope23/2
  Product7/1 -> Heading_angle1/1(v_vel)
  From29/1 -> EarthtoWind2/1(E_vec)
  From18/1 -> Mux4/5
  Demux3/3 -> Mux4/3
  Saturation/1 -> Trigonometric Function/1
  Dot Product1/1 -> Sum/2
  Demux3/2 -> Mux4/2
  Divide2/1 -> Product2/2  "a"
  Gain/1 -> Sum1/1
  Cos/1 -> Dot Product/2
  Divide3/1 -> Asin1/1
  Constant7/1 -> Product1/1
  Asin1/1 -> Saturation1/1
  Product1/1 -> Divide2/1
  Heading_angle1/1(n) -> Saturation/1
  Unit Delay lift/1 -> Divide3/2
  Constant15/1 -> Path_8_sim_v4/2(np_ahead)
  Path_8_sim_v4/6(dist_p) -> Scope5/1
  Sum/1 -> Sum1/2
  EarthtoWind2/1(W_vec) -> Vector Concatenate3/1  "VelocityW"
  Convert YPR-tantoe1/2(pitch) -> Scope2/2  "pitch"
  Constant1/1 -> Multiport Switch1/3, Multiport Switch1/4
  Saturation1/1 -> Scope18/1, Mux4/4
  Mux4/1 -> Convert YPR-tantoe1/1(input)
  Demux3/1 -> Mux4/1
  Multiport Switch1/1 -> Goto1/1
  Trigonometric Function1/1 -> Dot Product1/2
  Demux2/1 -> Terminator/1
  From1/1 -> Divide2/2
  Clock/1 -> Switch/2
  Vector Concatenate3/1 -> Product7/2
  From30/1 -> Product7/1
  From10/1 -> Cos/1, Trigonometric Function1/1
  From5/1 -> Multiport Switch1/1
  Demux2/2 -> Dot Product/1
  EarthtoWind3/1(W_vec) -> Path_8_sim_v4/1(a_posW)
  From20/1 -> Demux3/1
  Path_8_sim_v4/5(d_l1) -> Switch/1  "d_L1"
  From28/1 -> Product6/1
  Constant14/1 -> Vector Concatenate1/2
  Transpose1/1 -> Product6/2
  From9/1 -> EarthtoWind3/1(E_vec)
  Product2/1 -> Gain/1
  From19/1 -> Mux4/6
  Vector Concatenate1/1 -> Transpose1/1
  Product6/1 -> Heading_angle1/2(v_targ)  "TargetvecW"
  Sum1/1 -> Divide3/1
  Constant11/1 -> Switch/3
  Dot Product4/1 -> Product1/3
  Path_8_sim_v4/1(target_p) -> Vector Concatenate1/1
  Switch/1 -> Multiport Switch1/2
  Path_8_sim_v4/2(closest_p) -> To Workspace1/1, Scope6/1
  traction/3(alpha_path) -> [Alpha_path]
  traction/2(crossTrackErr) -> Crosstrackerr/1
  traction/1(desired_roll_tract) -> Multiport Switch2/4, Multiport Switch2/2
  [state] -> Equal/1
  Retraction/2(desired_descent_angle) -> Angle_of_Attack/1(desired_descent_angle)
  Angle_of_Attack/1(desired_alpha) -> des_alpha/1
  [state] -> Angle_of_Attack/2(flightState)
  roll pitch yaw/1 -> Convert YPR-e_to_tan/2(kite_angles)
  Convert YPR-e_to_tan/1(roll_tang) -> traction/3(roll_tang)
  Convert YPR-e_to_tan/4(actual_roll) -> actual roll/1
  Convert YPR-e_to_tan/2(pitch_tang) -> traction/4(pitch_tang)
  Convert YPR-e_to_tan/3(yaw_tang) -> actual yaw/1, traction/5(yaw_tang)
  traction/4(target_spath) -> [spath_target]

== system simL0_multiPath/Controls/AttitudeControl ==
  desired roll : Inport
  actual roll : Inport  Port=2
  desired alpha : Inport  Port=3
  actual alpha : Inport  Port=4
  F_state : Inport  Port=5
  "ang_desce_actual " : Inport  Port=6
  actual yaw : Inport  Port=7
  desired yaw : Inport  Port=8
  Pitch : Subsystem
  Roll : Subsystem
  Yaw : Subsystem  Commented=on
  roll rate desired : Outport  VectorParamsAs1DForOutWhenUnconnected=off
  pitch rate desired : Outport  Port=2  VectorParamsAs1DForOutWhenUnconnected=off
  yaw rate desired : Outport  Port=3  VectorParamsAs1DForOutWhenUnconnected=off
  tag scope: F_state=global
  wires:
  F_state/1 -> [F_state]
  desired alpha/1 -> Pitch/1(desiredAlpha)
  actual alpha/1 -> Pitch/2(actualAlpha)
  "ang_desce_actual "/1 -> Pitch/3(actualDescentAngle)
  Pitch/1(desiredPitchRate) -> pitch rate desired/1
  desired roll/1 -> Roll/1(desiredRoll)
  actual roll/1 -> Roll/2(actualRoll)
  Roll/1(desiredRollRate) -> roll rate desired/1
  actual yaw/1 -> Yaw/2(actualYaw)
  desired yaw/1 -> Yaw/1(desiredYaw)
  Yaw/1(desiredyawRate) -> yaw rate desired/1

== system simL0_multiPath/Controls/RatesControl ==
  note: positive flap angles result in negative yaw moment
  roll rate desired : Inport
  pitch rate desired : Inport  Port=2
  yaw rate desired : Inport  Port=3
  airspeed : Inport  Port=4
  p-q-r : Inport  Port=5
  Add : Sum
  Constant4 : Constant  Value=0
  Demux1 : Demux  Outputs=3
  Demux2 : Demux  Outputs=3
  Gain1 : Gain  Gain=actuatorLimit.deflectionAileron
  Gain2 : Gain  Gain=-actuatorLimit.deflectionElevator
  Gain3 : Gain  Commented=on  Gain=-actuatorLimit.deflectionRudder
  Magnitude Squared : Math  Operator=square
  Magnitude Squared1 : Math  Operator=square
  Terminator : Terminator  Commented=on
  Terminator2 : Terminator
  rate controller : Subsystem
  sqrt : Math  Operator=sqrt  SignedPower=on
  aileron deflection : Outport  VectorParamsAs1DForOutWhenUnconnected=off
  elevator deflection : Outport  Port=2  VectorParamsAs1DForOutWhenUnconnected=off
  rudder deflection : Outport  Port=3  VectorParamsAs1DForOutWhenUnconnected=off
  wires:
  Gain1/1 -> aileron deflection/1  "aileron"
  Demux2/3 -> rate controller/6(r)  "r"
  Gain2/1 -> elevator deflection/1  "elevator"
  sqrt/1 -> rate controller/7(V_T)  "V_T"
  airspeed/1 -> Demux1/1
  yaw rate desired/1 -> rate controller/3(r_c)
  rate controller/2(pitch) -> Gain2/1
  rate controller/3(yaw) -> Gain3/1
  Demux2/2 -> rate controller/5(q)  "q"
  Demux2/1 -> rate controller/4(p)  "p"
  Magnitude Squared/1 -> Add/1
  Add/1 -> sqrt/1
  rate controller/1(roll) -> Gain1/1
  Demux1/3 -> Magnitude Squared1/1
  Demux1/1 -> Magnitude Squared/1
  p-q-r/1 -> Demux2/1
  Demux1/2 -> Terminator2/1
  roll rate desired/1 -> rate controller/1(p_c)
  pitch rate desired/1 -> rate controller/2(q_c)
  Constant4/1 -> rudder deflection/1
  Gain3/1 -> Terminator/1  "rudder"
  Magnitude Squared1/1 -> Add/2

== system simL0_multiPath/Environment_WindModel/wind_field_calc ==
  Altitude : Inport
  Base_windspeed : Inport  Port=2
  1-D Lookup Table : Lookup_n-D  NumberOfTableDimensions=1  BreakpointsForDimension1=ENVMT.wind_height  Table=ENVMT.wind_data  InternalRulePriority=Speed  RndMeth=Simplest
  Product2 : Product  InputSameDT=on  SaturateOnIntegerOverflow=on  OutDataTypeStr=Inherit: Same as first input
  Reshape : Reshape  OutputDimensionality=Column vector (2-D)
  Saturation : Saturate  UpperLimit=ENVMT.height_max  LowerLimit=ENVMT.wind_height(1)
  Windspeed_altitude : Outport
  wires:
  Product2/1 -> Reshape/1  "referencce location"
  1-D Lookup Table/1 -> Product2/1
  Reshape/1 -> Windspeed_altitude/1
  Base_windspeed/1 -> Product2/2
  Saturation/1 -> 1-D Lookup Table/1  "ijmuiden"
  Altitude/1 -> Saturation/1

== system simL0_multiPath/GroundStationMegAWES/ New_Winch_controller_Traction ==
  note: Flight state is in traction or Transition
  traction_torque_cmd : Inport
  torque_cmd : Inport  Port=2
  Input : Inport  Port=3
  Compare To Constant : simulink/Logic and Bit Operations/Compare To Constant  relop===  const=1  OutDataTypeStr=boolean
  Scope : Scope
  Switch : Switch  Criteria=u2 > Threshold  SaturateOnIntegerOverflow=off  InputSameDT=off
  control_moments : Outport
  wires:
  traction_torque_cmd/1 -> Switch/1
  Input/1 -> Compare To Constant/1
  torque_cmd/1 -> Switch/3
  Switch/1 -> control_moments/1
  Compare To Constant/1 -> Switch/2, Scope/1
